simulink library "lib_accessory"  (Simulink 4.1.1)
undefined symbols (not defined in the file): acc_dcdc_eff, acc_elec_eff, acc_elec_efficiency, acc_elec_pwr, acc_mech_eff, acc_mech_pwr, acc_mech_trq, acc_sindafile, amb_tmp, cyc_mph, ess_on, fc_on, fd_ratio, gb_ratio, load_on, map_spd, max_pwr, tc_gc_to_fc_ratio, time_step, vc_idle_bool, vc_idle_spd, vinf, wh_radius
libraries: lib_accessory x47, lib_cosimulation x29, lib_outputs x11, simulink3 x4, sub_lib_models x2
(part 3 of 3)

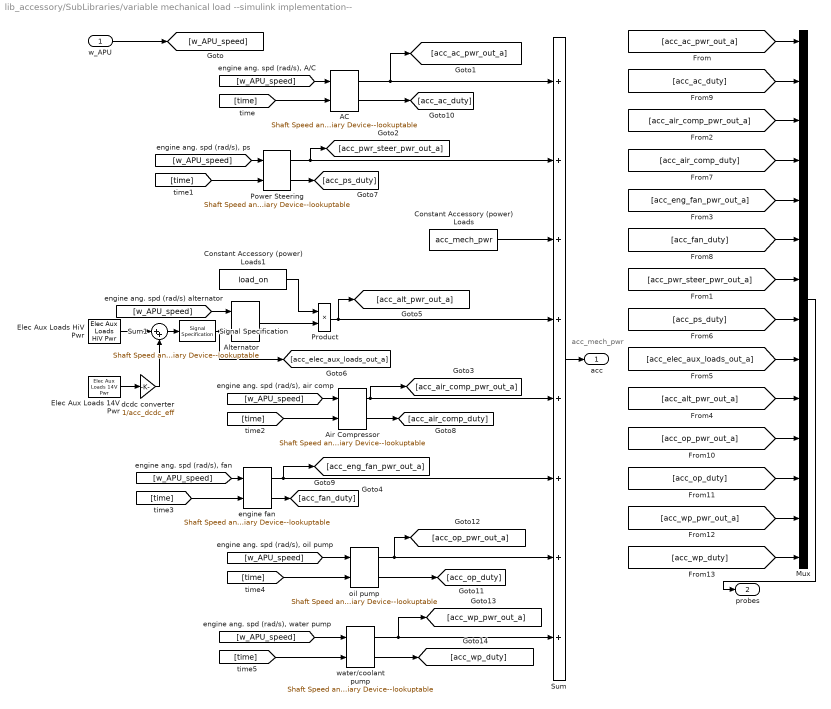
== system lib_accessory/SubLibraries/variable mechanical load --simulink implementation-- ==
  note: acc_mech_pwr
  w_APU : Inport  Port=1  LatchInput=off
  AC : lib_accessory/SubLibraries/Shaft Speed and Time Loaded Auxiliary Device--lookuptable  fname=acc_ac_init  acc_duty=acc_ac_dutycycle
  Air Compressor : lib_accessory/SubLibraries/Shaft Speed and Time Loaded Auxiliary Device--lookuptable  fname=acc_abc_init  acc_duty=acc_abc_dutycycle
  Alternator : lib_accessory/SubLibraries/Shaft Speed and Actual Load Auxiliary Device--lookuptable  conv_eff=acc_acdc_inverter_eff  fname=acc_alt_init
  Constant Accessory (power) Loads : Constant  Value=acc_mech_pwr
  Constant Accessory (power) Loads1 : Constant  Value=load_on
  Elec Aux Loads 14V Pwr : lib_accessory/Elec Aux Loads 14V Pwr
      settings: RTWFcnNameOpts=Auto  RTWFileNameOpts=Auto
  Elec Aux Loads HiV Pwr : lib_accessory/Elec Aux Loads HiV Pwr
      settings: RTWFcnNameOpts=Auto  RTWFileNameOpts=Auto
  Mux : Mux  Inputs=14
  Power Steering : lib_accessory/SubLibraries/Shaft Speed and Time Loaded Auxiliary Device--lookuptable  fname=acc_ps_init  acc_duty=acc_ps_dutycycle
  Product : Product  Inputs=2  Multiplication=Element-wise(.*)  SaturateOnIntegerOverflow=on
  Signal Specification : simulink3/Signals & Systems/Signal Specification  D=1  Ts=-1  DataType=auto
  Sum : Sum  Inputs=++++++++  SaturateOnIntegerOverflow=on
  Sum1 : Sum  Inputs=|++  SaturateOnIntegerOverflow=on
  dcdc converter : Gain  Gain=1/acc_dcdc_eff  Multiplication=Element-wise(K.*u)  SaturateOnIntegerOverflow=on
  engine fan : lib_accessory/SubLibraries/Shaft Speed and Time Loaded Auxiliary Device--lookuptable  fname=acc_ef_init  acc_duty=acc_ef_dutycycle
  oil pump : lib_accessory/SubLibraries/Shaft Speed and Time Loaded Auxiliary Device--lookuptable  fname=acc_op_init  acc_duty=acc_op_dutycycle
  water/coolant pump : lib_accessory/SubLibraries/Shaft Speed and Time Loaded Auxiliary Device--lookuptable  fname=acc_wp_init  acc_duty=acc_wp_dutycycle
  acc : Outport  Port=1
  probes : Outport  Port=2
  wires:
  [time] -> AC/2
  [w_APU_speed] -> AC/1
  AC/2 -> [acc_ac_duty]
  AC/1 -> Sum/1, [acc_ac_pwr_out_a]
  Constant Accessory (power) Loads/1 -> Sum/3
  Sum/1 -> acc/1
  [w_APU_speed] -> Alternator/1
  Air Compressor/2 -> [acc_air_comp_duty]
  Air Compressor/1 -> Sum/5, [acc_air_comp_pwr_out_a]
  [w_APU_speed] -> Air Compressor/1
  [time] -> Air Compressor/2
  oil pump/1 -> [acc_op_pwr_out_a], Sum/7
  oil pump/2 -> [acc_op_duty]
  [time] -> oil pump/2
  [w_APU_speed] -> oil pump/1
  engine fan/2 -> [acc_fan_duty]
  [time] -> engine fan/2
  engine fan/1 -> Sum/6, [acc_eng_fan_pwr_out_a]
  [w_APU_speed] -> engine fan/1
  Power Steering/2 -> [acc_ps_duty]
  [w_APU_speed] -> Power Steering/1
  [time] -> Power Steering/2
  Power Steering/1 -> Sum/2, [acc_pwr_steer_pwr_out_a]
  w_APU/1 -> [w_APU_speed]
  Elec Aux Loads 14V Pwr/1 -> dcdc converter/1
  Signal Specification/1 -> Alternator/2, [acc_elec_aux_loads_out_a]
  [acc_ac_pwr_out_a] -> Mux/1
  Product/1 -> Sum/4, [acc_alt_pwr_out_a]
  Constant Accessory (power) Loads1/1 -> Product/1
  Alternator/1 -> Product/2
  Mux/1 -> probes/1
  water/coolant pump/1 -> Sum/8, [acc_wp_pwr_out_a]
  [time] -> water/coolant pump/2
  [w_APU_speed] -> water/coolant pump/1
  water/coolant pump/2 -> [acc_wp_duty]
  [acc_ac_duty] -> Mux/2
  [acc_air_comp_pwr_out_a] -> Mux/3
  [acc_air_comp_duty] -> Mux/4
  [acc_eng_fan_pwr_out_a] -> Mux/5
  [acc_fan_duty] -> Mux/6
  [acc_pwr_steer_pwr_out_a] -> Mux/7
  [acc_ps_duty] -> Mux/8
  [acc_elec_aux_loads_out_a] -> Mux/9
  [acc_alt_pwr_out_a] -> Mux/10
  [acc_op_pwr_out_a] -> Mux/11
  [acc_op_duty] -> Mux/12
  [acc_wp_pwr_out_a] -> Mux/13
  [acc_wp_duty] -> Mux/14
  Sum1/1 -> Signal Specification/1
  Elec Aux Loads HiV Pwr/1 -> Sum1/1
  dcdc converter/1 -> Sum1/2

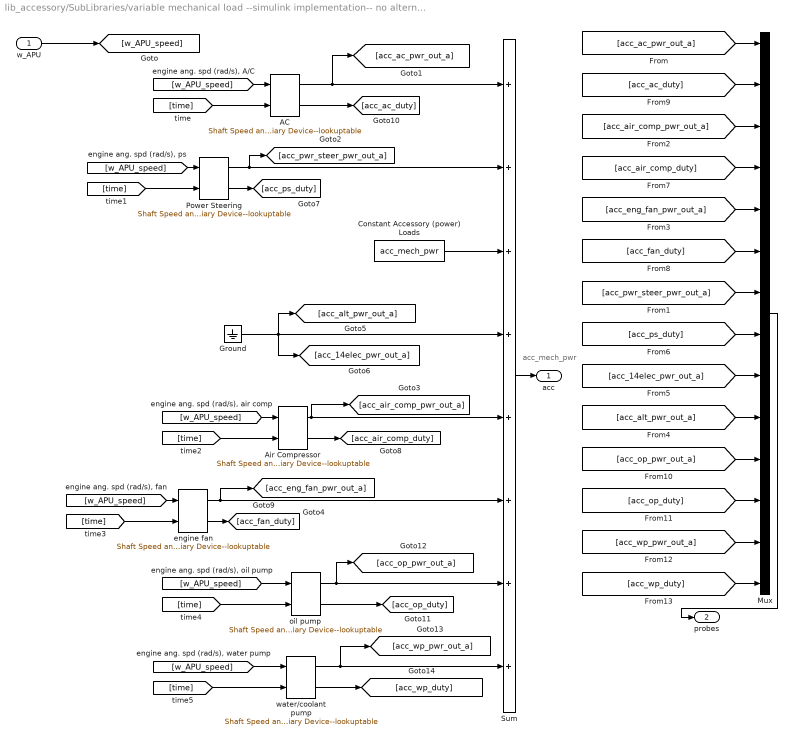
== system lib_accessory/SubLibraries/variable mechanical load --simulink implementation-- no alternator ==
  note: acc_mech_pwr
  w_APU : Inport  Port=1  LatchInput=off
  AC : lib_accessory/SubLibraries/Shaft Speed and Time Loaded Auxiliary Device--lookuptable  fname=acc_ac_init  acc_duty=acc_ac_dutycycle
  Air Compressor : lib_accessory/SubLibraries/Shaft Speed and Time Loaded Auxiliary Device--lookuptable  fname=acc_abc_init  acc_duty=acc_abc_dutycycle
  Constant Accessory (power) Loads : Constant  Value=acc_mech_pwr
  Ground : Ground
  Mux : Mux  Inputs=14
  Power Steering : lib_accessory/SubLibraries/Shaft Speed and Time Loaded Auxiliary Device--lookuptable  fname=acc_ps_init  acc_duty=acc_ps_dutycycle
  Sum : Sum  Inputs=++++++++  SaturateOnIntegerOverflow=on
  engine fan : lib_accessory/SubLibraries/Shaft Speed and Time Loaded Auxiliary Device--lookuptable  fname=acc_ef_init  acc_duty=acc_ef_dutycycle
  oil pump : lib_accessory/SubLibraries/Shaft Speed and Time Loaded Auxiliary Device--lookuptable  fname=acc_op_init  acc_duty=acc_op_dutycycle
  water/coolant pump : lib_accessory/SubLibraries/Shaft Speed and Time Loaded Auxiliary Device--lookuptable  fname=acc_wp_init  acc_duty=acc_wp_dutycycle
  acc : Outport  Port=1
  probes : Outport  Port=2
  wires:
  [time] -> AC/2
  [w_APU_speed] -> AC/1
  AC/2 -> [acc_ac_duty]
  AC/1 -> Sum/1, [acc_ac_pwr_out_a]
  Constant Accessory (power) Loads/1 -> Sum/3
  Sum/1 -> acc/1
  Air Compressor/2 -> [acc_air_comp_duty]
  Air Compressor/1 -> Sum/5, [acc_air_comp_pwr_out_a]
  [w_APU_speed] -> Air Compressor/1
  [time] -> Air Compressor/2
  oil pump/1 -> [acc_op_pwr_out_a], Sum/7
  oil pump/2 -> [acc_op_duty]
  [time] -> oil pump/2
  [w_APU_speed] -> oil pump/1
  engine fan/2 -> [acc_fan_duty]
  [time] -> engine fan/2
  engine fan/1 -> Sum/6, [acc_eng_fan_pwr_out_a]
  [w_APU_speed] -> engine fan/1
  Power Steering/2 -> [acc_ps_duty]
  [w_APU_speed] -> Power Steering/1
  [time] -> Power Steering/2
  Power Steering/1 -> Sum/2, [acc_pwr_steer_pwr_out_a]
  w_APU/1 -> [w_APU_speed]
  [acc_ac_pwr_out_a] -> Mux/1
  Ground/1 -> Sum/4, [acc_alt_pwr_out_a], [acc_14elec_pwr_out_a]
  Mux/1 -> probes/1
  water/coolant pump/1 -> Sum/8, [acc_wp_pwr_out_a]
  [time] -> water/coolant pump/2
  [w_APU_speed] -> water/coolant pump/1
  water/coolant pump/2 -> [acc_wp_duty]
  [acc_ac_duty] -> Mux/2
  [acc_air_comp_pwr_out_a] -> Mux/3
  [acc_air_comp_duty] -> Mux/4
  [acc_eng_fan_pwr_out_a] -> Mux/5
  [acc_fan_duty] -> Mux/6
  [acc_pwr_steer_pwr_out_a] -> Mux/7
  [acc_ps_duty] -> Mux/8
  [acc_14elec_pwr_out_a] -> Mux/9
  [acc_alt_pwr_out_a] -> Mux/10
  [acc_op_pwr_out_a] -> Mux/11
  [acc_op_duty] -> Mux/12
  [acc_wp_pwr_out_a] -> Mux/13
  [acc_wp_duty] -> Mux/14

== system lib_accessory/Development/Electrical Accessory Loads <acc>/Accessory SDO ==
  data bus : Inport  Port=1  LatchInput=off
  Demux : Demux  Outputs=3  BusSelectionMode=off
  To Workspace : ToWorkspace  VariableName=acc_elec_pwr_r  SampleTime=-1  SaveFormat=Array
  To Workspace3 : ToWorkspace  VariableName=acc_elec_pwr_a  SampleTime=-1  SaveFormat=Array
  To Workspace4 : ToWorkspace  VariableName=acc_elec_pwr_est  SampleTime=-1  SaveFormat=Array
  electrical power logging : lib_accessory/SubLibraries/electrical power logging  eff=acc_mech_eff
  wires:
  data bus/1 -> Demux/1
  Demux/1 -> To Workspace/1
  Demux/2 -> To Workspace3/1, electrical power logging/1
  Demux/3 -> To Workspace4/1

== system lib_accessory/Development/Electrical Accessory Loads <acc>/Block NOTES ==
  note: In terms of an interface, the model assumes electrical power generated from
      | a powersource (or powersources)
      |
      | This model takes in requested driveline electrical power output requests and
      | augments power to account for electrically driven accessories.
      |
      | The power passed along down to the driveline is only power to move the
      | vehicle.
  note: This is the electrical auxiliary loads model.

== system lib_accessory/Development/Electrical Accessory Loads <acc>/backward model ==
  note: Pwr, W, powersource out
  note: P, W, for driveline
  note: Power Electrical
      | Accessory
      | (W)
  pwr_in : Inport  Port=1  LatchInput=off
  Sum : Sum  Inputs=|++  SaturateOnIntegerOverflow=on
  electrical accessories (W) : Subsystem  BlockChoice=Electrical Accessories: Time Variable
      settings: AttributesFormatString=%<BlockChoice>  TemplateBlock=lib_accessory/electrical accessories (W)  MemberBlocks=Electrical Accessories: Constant,Electrical Accessories: Time Variable  RTWFcnNameOpts=Auto  RTWFileNameOpts=Auto
      mask Display: image(imread('bdi_acc_elec.bmp'))
  elec_out : Outport  Port=1
  elec_acc_out : Outport  Port=2
  wires:
  electrical accessories (W)/1(P_elec_acc) -> elec_acc_out/1, Sum/2
  Sum/1 -> elec_out/1
  pwr_in/1 -> Sum/1

== system lib_accessory/Development/Electrical Accessory Loads <acc>/forward model ==
  note: Power to driveline
  note: Power Available
  note: electric
      | accessory
      | power (W)
  pwr_in : Inport  Port=1  LatchInput=off
  Sum : Sum  Inputs=|+-  SaturateOnIntegerOverflow=on
  electrical accessories (W) : Subsystem  BlockChoice=Electrical Accessories: Time Variable
      settings: AttributesFormatString=%<BlockChoice>  TemplateBlock=lib_accessory/electrical accessories (W)  MemberBlocks=Electrical Accessories: Constant,Electrical Accessories: Time Variable  RTWFcnNameOpts=Auto  RTWFileNameOpts=Auto
      mask Display: image(imread('bdi_acc_elec.bmp'))
  pwr_out : Outport  Port=1
  acc_pwr_out : Outport  Port=2
  wires:
  electrical accessories (W)/1(P_elec_acc) -> acc_pwr_out/1, Sum/2
  Sum/1 -> pwr_out/1
  pwr_in/1 -> Sum/1

== system lib_accessory/Development/Mechanical Accessory Loads <acc>/Accessory SDO ==
  data bus : Inport  Port=1  LatchInput=off
  Demux : Demux  Outputs=5  BusSelectionMode=off
  To Workspace : ToWorkspace  VariableName=acc_mech_trq_r  SampleTime=-1  SaveFormat=Array
  To Workspace1 : ToWorkspace  VariableName=acc_mech_pwr_a  SampleTime=-1  SaveFormat=Array
  To Workspace2 : ToWorkspace  VariableName=acc_mech_trq_est  SampleTime=-1  SaveFormat=Array
  To Workspace3 : ToWorkspace  VariableName=acc_mech_pwr_r  SampleTime=-1  SaveFormat=Array
  To Workspace4 : ToWorkspace  VariableName=acc_mech_trq_a  SampleTime=-1  SaveFormat=Array
  mechanical power logging : lib_accessory/SubLibraries/mechanical power logging  eff=acc_mech_eff
  wires:
  data bus/1 -> Demux/1
  Demux/4 -> mechanical power logging/1, To Workspace1/1
  Demux/1 -> To Workspace/1
  Demux/2 -> To Workspace3/1
  Demux/3 -> To Workspace4/1
  Demux/5 -> To Workspace2/1

== system lib_accessory/Development/Mechanical Accessory Loads <acc>/Block NOTES ==
  note: This is the mechanical auxiliary loads model.
  note: In terms of an interface, the model assumes belt-driven mechanical loads
      | that run off of a prime mover shaft (e.g., engine shaft)
      |
      | This model takes in requested driveline torque and speed requests and
      | augments torque due to belt driven accessories.
      |
      | The torque passed along down to the driveline is only torque to move the
      | vehicle.

== system lib_accessory/Development/Mechanical Accessory Loads <acc>/backward model ==
  note: w_apu, rad/s
  note: T, Nm, accessory
  note: T, Nm, driveline
  note: T, Nm, shaft out
  note: Power, W, input to accessory
  trq_in : Inport  Port=1  LatchInput=off
  spd_in : Inport  Port=2  LatchInput=off
  Sum : Sum  Inputs=|++  SaturateOnIntegerOverflow=on
  mechanical accessories (Nm) : Subsystem  BlockChoice=Mechanical Accessories: Const Mech Var Elect
      settings: AttributesFormatString=%<BlockChoice>  TemplateBlock=lib_accessory/mechanical accessories (Nm)  MemberBlocks=Mechanical Accessories: Const Mech Var Elect,Mechanical Accessories: Constant Load No Alternator,Mechanical Accessories: Constant Mechanical & Electrical,Mechanical Accessories: Speed Dependant No Alternator,Mechanical Accessories: Speed Dependant and Variable Electrical  RTWFcnNameOpts=Auto  RTWFileNameOpts=Auto
      mask Display: image(imread('bdi_acc_pic.bmp'))
  trq_out : Outport  Port=1
  spd_out : Outport  Port=2
  acc_mech_trq_r : Outport  Port=3
  acc_mech_pwr_r : Outport  Port=4
  wires:
  spd_in/1 -> spd_out/1, mechanical accessories (Nm)/1(w_APU)
  mechanical accessories (Nm)/1(T_acc) -> acc_mech_trq_r/1, Sum/2
  trq_in/1 -> Sum/1
  Sum/1 -> trq_out/1
  mechanical accessories (Nm)/2(P_mech_acc) -> acc_mech_pwr_r/1

== system lib_accessory/Development/Mechanical Accessory Loads <acc>/estimated mechanical torque ==
  spd_in : Inport  Port=1  LatchInput=off
  mech pwr : Terminator
  mechanical accessories (Nm) : Subsystem  BlockChoice=Mechanical Accessories: Const Mech Var Elect
      settings: AttributesFormatString=%<BlockChoice>  TemplateBlock=lib_accessory/mechanical accessories (Nm)  MemberBlocks=Mechanical Accessories: Const Mech Var Elect,Mechanical Accessories: Constant Load No Alternator,Mechanical Accessories: Constant Mechanical & Electrical,Mechanical Accessories: Speed Dependant No Alternator,Mechanical Accessories: Speed Dependant and Variable Electrical  RTWFcnNameOpts=Auto  RTWFileNameOpts=Auto
      mask Display: image(imread('bdi_acc_pic.bmp'))
  trq_out : Outport  Port=1
  wires:
  spd_in/1 -> mechanical accessories (Nm)/1(w_APU)
  mechanical accessories (Nm)/2(P_mech_acc) -> mech pwr/1
  mechanical accessories (Nm)/1(T_acc) -> trq_out/1

== system lib_accessory/Development/Mechanical Accessory Loads <acc>/forward model ==
  note: w_apu, rad/s
  note: T, Nm, accessory
  note: T, Nm, driveline
  note: T, Nm, shaft out
  note: Power, W, input to accessory
  trq_in : Inport  Port=1  LatchInput=off
  spd_in : Inport  Port=2  LatchInput=off
  Sum : Sum  Inputs=|+-  SaturateOnIntegerOverflow=on
  mechanical accessories (Nm) : Subsystem  BlockChoice=Mechanical Accessories: Const Mech Var Elect
      settings: AttributesFormatString=%<BlockChoice>  TemplateBlock=lib_accessory/mechanical accessories (Nm)  MemberBlocks=Mechanical Accessories: Const Mech Var Elect,Mechanical Accessories: Constant Load No Alternator,Mechanical Accessories: Constant Mechanical & Electrical,Mechanical Accessories: Speed Dependant No Alternator,Mechanical Accessories: Speed Dependant and Variable Electrical  RTWFcnNameOpts=Auto  RTWFileNameOpts=Auto
      mask Display: image(imread('bdi_acc_pic.bmp'))
  trq_out : Outport  Port=1
  spd_out : Outport  Port=2
  acc_mech_trq_a : Outport  Port=3
  acc_mech_pwr_a : Outport  Port=4
  wires:
  spd_in/1 -> spd_out/1, mechanical accessories (Nm)/1(w_APU)
  mechanical accessories (Nm)/1(T_acc) -> acc_mech_trq_a/1, Sum/2
  trq_in/1 -> Sum/1
  Sum/1 -> trq_out/1
  mechanical accessories (Nm)/2(P_mech_acc) -> acc_mech_pwr_a/1

== system lib_accessory/Elec Aux Loads HiV Pwr/Starter/Starter ==
  14 V : Constant  Value=vinf.AuxLoads.Starter.HiV
  Hit  Crossing : HitCross  HitCrossingOffset=0  HitCrossingDirection=rising  ShowOutputPort=on
  Memory : Memory  X0=fc_on  InheritSampleTime=off
      settings: RTWStateStorageClass=Auto
  On : Constant  Value=vinf.AuxLoads.Starter.On
  Product1 : Product  Inputs=4  Multiplication=Element-wise(.*)  SaturateOnIntegerOverflow=on
  Subsystem : Subsystem
      settings: RTWFcnNameOpts=Auto  RTWFileNameOpts=Auto
  Starter_OnOff_Control : Outport  Port=1
  wires:
  14 V/1 -> Product1/2
  Subsystem/1(Out1) -> Product1/3
  Product1/1 -> Starter_OnOff_Control/1
  On/1 -> Product1/1
  [key_on] -> Product1/4
  [time] -> Subsystem/2(In2)
  [engine_on] -> Memory/1
  Hit  Crossing/1 -> Subsystem/1(In1)
  Memory/1 -> Hit  Crossing/1

== system lib_accessory/Electrical Accessory Loads v2 <acc>/backward model/electrical accessories (W) ==
  Electrical Accessories: Time Variable : lib_accessory/Electrical Accessories: Time Variable
  P_elec_acc : Outport  Port=1
  wires:
  Electrical Accessories: Time Variable/1 -> P_elec_acc/1

== system lib_accessory/Mechanical Accessory Loads v2 <acc>/backward model/mechanical accessories (Nm) ==
  w_APU : Inport  Port=1  LatchInput=off
  Mechanical Accessories: Const Mech Var Elect : lib_accessory/Mechanical Accessories: Const Mech Var Elect
  T_acc : Outport  Port=1
  P_mech_acc : Outport  Port=2
  probes : Outport  Port=3
  wires:
  w_APU/1 -> Mechanical Accessories: Const Mech Var Elect/1
  Mechanical Accessories: Const Mech Var Elect/1 -> T_acc/1
  Mechanical Accessories: Const Mech Var Elect/2 -> P_mech_acc/1
  Mechanical Accessories: Const Mech Var Elect/3 -> probes/1

== system lib_accessory/Saber Dual Voltage Cosim/saber dv acc/DV cosim output gotos ==
  In1 : Inport  Port=1  LatchInput=off
  Demux : Demux  Outputs=[4 4 4 2 2 30 12]  BusSelectionMode=off
  Saber_ess2_outputs : Subsystem  BlockChoice=Saber_rint2
      settings: AttributesFormatString=%<BlockChoice>  TemplateBlock=lib_outputs/Saber_ess2_outputs  MemberBlocks=Saber_pb2,Saber_rint2  RTWFcnNameOpts=Auto  RTWFileNameOpts=Auto
  Saber_ess_outputs : Subsystem  BlockChoice=Saber_rint
      settings: AttributesFormatString=%<BlockChoice>  TemplateBlock=lib_outputs/Saber_ess_outputs  MemberBlocks=Saber_pb,Saber_rint  RTWFcnNameOpts=Auto  RTWFileNameOpts=Auto
  saber acc 14v output gotos : lib_outputs/saber acc 14v output gotos
      settings: RTWFcnNameOpts=Auto  RTWFileNameOpts=Auto
  saber acc HiV output gotos : lib_outputs/saber acc HiV output gotos
      settings: RTWFcnNameOpts=Auto  RTWFileNameOpts=Auto
  saber acc additional outputs : lib_outputs/saber acc additional outputs
      settings: RTWFcnNameOpts=Auto  RTWFileNameOpts=Auto
  saber dcdc output gotos : lib_outputs/saber dcdc output gotos
      settings: RTWFcnNameOpts=Auto  RTWFileNameOpts=Auto
  saber gc output gotos : lib_outputs/saber gc output gotos
      settings: RTWFcnNameOpts=Auto  RTWFileNameOpts=Auto
  Out1 : Outport  Port=1
  wires:
  Demux/3 -> Saber_ess2_outputs/1(In1)
  Demux/2 -> Saber_ess_outputs/1(In1)
  In1/1 -> Demux/1
  Demux/1 -> saber gc output gotos/1
  Demux/4 -> saber dcdc output gotos/1
  saber gc output gotos/1 -> Out1/1
  Demux/6 -> saber acc 14v output gotos/1
  Demux/7 -> saber acc HiV output gotos/1
  Demux/5 -> saber acc additional outputs/1

== system lib_accessory/Saber Dual Voltage Cosim/saber dv acc/Engine Info ==
  w_apu : Inport  Port=1  LatchInput=off
  Constant : Constant  Value=0
  Enabled Subsystem : Subsystem  TreatAsAtomicUnit=on
      settings: RTWFcnNameOpts=Auto  RTWFileNameOpts=Auto
  IC : InitialCondition  Value=time_step
  Matrix Concatenation1 : S-Function  FunctionName=smatrxcat  Parameters=numInports,catMethod  PortCounts=[]  SFunctionModules=''  mask(Matrix Concatenation){numInports=6, catMethod=Horizontal}
      mask prompts: numInports "Number of inputs:"; catMethod "Concatenation method:"
      mask help: Perform horizontal or vertical concatenation. 1-D vector input signals are treated as column vectors, i.e., [Mx1] matrices. The output is always a matrix.
      mask init:
      | xy = matrxcatmask('icon');
      mask StyleString: edit,popup(Horizontal|Vertical)
      mask Display:
      | plot(xy.x,xy.y);
      | text(0.15,0.86,xy.label);
  Memory1 : Memory  X0=.001  InheritSampleTime=on
      settings: RTWStateStorageClass=Auto
  Memory2 : Memory  X0=80  InheritSampleTime=on
      settings: RTWStateStorageClass=Auto
  Relational Operator : RelationalOperator  Operator===
  Saturation : Saturate  UpperLimit=inf  LowerLimit=.001  LinearizeAsGain=on
  pulley ratio : Gain  Gain=tc_gc_to_fc_ratio  Multiplication=Element-wise(K.*u)  SaturateOnIntegerOverflow=on
  "rad/s -> rpm1" : Gain  Gain=60/(2*pi)  Multiplication=Element-wise(K.*u)  SaturateOnIntegerOverflow=on
  RPM : Outport  Port=1
  wires:
  Relational Operator/1 -> Enabled Subsystem/Enable
  [time] -> Relational Operator/2
  Enabled Subsystem/1(Out1) -> Matrix Concatenation1/2
  Memory2/1 -> Matrix Concatenation1/4
  Matrix Concatenation1/1 -> RPM/1
  IC/1 -> Matrix Concatenation1/5
  Saturation/1 -> Memory1/1
  [time] -> Saturation/1
  Memory1/1 -> Matrix Concatenation1/3
  [time] -> IC/1
  Constant/1 -> Relational Operator/1, Matrix Concatenation1/1
  w_apu/1 -> "rad/s -> rpm1"/1  "w_apu"
  "rad/s -> rpm1"/1 -> pulley ratio/1
  pulley ratio/1 -> Enabled Subsystem/1(In1), Matrix Concatenation1/6, Memory2/1

== system lib_accessory/Saber Dual Voltage Cosim/saber dv acc/Model Data In ==
  Aux Loads 14V and 42V : Subsystem
      settings: RTWFcnNameOpts=Auto  RTWFileNameOpts=Auto
  DC/DC converter : lib_cosimulation/DC//DC converter
      settings: RTWFcnNameOpts=Auto  RTWFileNameOpts=Auto
  Generator : lib_cosimulation/Generator
      settings: RTWFcnNameOpts=Auto  RTWFileNameOpts=Auto
  Matrix Concatenation1 : S-Function  FunctionName=smatrxcat  Parameters=numInports,catMethod  PortCounts=[]  SFunctionModules=''  mask(Matrix Concatenation){numInports=6, catMethod=Horizontal}
      mask prompts: numInports "Number of inputs:"; catMethod "Concatenation method:"
      mask help: Perform horizontal or vertical concatenation. 1-D vector input signals are treated as column vectors, i.e., [Mx1] matrices. The output is always a matrix.
      mask init:
      | xy = matrxcatmask('icon');
      mask StyleString: edit,popup(Horizontal|Vertical)
      mask Display:
      | plot(xy.x,xy.y);
      | text(0.15,0.86,xy.label);
  Regulator : lib_cosimulation/Regulator
      settings: RTWFcnNameOpts=Auto  RTWFileNameOpts=Auto
  ess param inputs : Subsystem  BlockChoice=Rint
      settings: AttributesFormatString=%<BlockChoice>  TemplateBlock=lib_cosimulation/ess param inputs  MemberBlocks=Rint,Saber lib pb  RTWFcnNameOpts=Auto  RTWFileNameOpts=Auto
  ess2 param inputs : Subsystem  BlockChoice=Rint2
      settings: AttributesFormatString=%<BlockChoice>  TemplateBlock=lib_cosimulation/ess2 param inputs  MemberBlocks=Rint2,Saber lib pb2  RTWFcnNameOpts=Auto  RTWFileNameOpts=Auto
  Out1 : Outport  Port=1
  wires:
  Aux Loads 14V and 42V/1(Out1) -> Matrix Concatenation1/1
  Regulator/1 -> Matrix Concatenation1/4
  Matrix Concatenation1/1 -> Out1/1
  Generator/1 -> Matrix Concatenation1/2
  DC/DC converter/1 -> Matrix Concatenation1/3
  ess param inputs/1(Out1) -> Matrix Concatenation1/5
  ess2 param inputs/1(Out1) -> Matrix Concatenation1/6

== system lib_accessory/Saber Single Voltage Cosim/saber sv acc/Engine Info ==
  w_apu : Inport  Port=1  LatchInput=off
  Constant : Constant  Value=0
  Enabled Subsystem : Subsystem  TreatAsAtomicUnit=on
      settings: RTWFcnNameOpts=Auto  RTWFileNameOpts=Auto
  IC : InitialCondition  Value=time_step
  Matrix Concatenation1 : S-Function  FunctionName=smatrxcat  Parameters=numInports,catMethod  PortCounts=[]  SFunctionModules=''  mask(Matrix Concatenation){numInports=6, catMethod=Horizontal}
      mask prompts: numInports "Number of inputs:"; catMethod "Concatenation method:"
      mask help: Perform horizontal or vertical concatenation. 1-D vector input signals are treated as column vectors, i.e., [Mx1] matrices. The output is always a matrix.
      mask init:
      | xy = matrxcatmask('icon');
      mask StyleString: edit,popup(Horizontal|Vertical)
      mask Display:
      | plot(xy.x,xy.y);
      | text(0.15,0.86,xy.label);
  Memory1 : Memory  X0=.001  InheritSampleTime=on
      settings: RTWStateStorageClass=Auto
  Memory2 : Memory  X0=80  InheritSampleTime=on
      settings: RTWStateStorageClass=Auto
  Relational Operator : RelationalOperator  Operator===
  Saturation : Saturate  UpperLimit=inf  LowerLimit=.001  LinearizeAsGain=on
  pulley ratio : Gain  Gain=tc_gc_to_fc_ratio  Multiplication=Element-wise(K.*u)  SaturateOnIntegerOverflow=on
  "rad/s -> rpm1" : Gain  Gain=60/(2*pi)  Multiplication=Element-wise(K.*u)  SaturateOnIntegerOverflow=on
  RPM : Outport  Port=1
  wires:
  Relational Operator/1 -> Enabled Subsystem/Enable
  [time] -> Relational Operator/2
  Enabled Subsystem/1(Out1) -> Matrix Concatenation1/2
  Memory2/1 -> Matrix Concatenation1/4
  Matrix Concatenation1/1 -> RPM/1
  IC/1 -> Matrix Concatenation1/5
  Saturation/1 -> Memory1/1
  [time] -> Saturation/1
  Memory1/1 -> Matrix Concatenation1/3
  [time] -> IC/1
  Constant/1 -> Relational Operator/1, Matrix Concatenation1/1
  w_apu/1 -> "rad/s -> rpm1"/1  "w_apu"
  "rad/s -> rpm1"/1 -> pulley ratio/1
  pulley ratio/1 -> Enabled Subsystem/1(In1), Matrix Concatenation1/6, Memory2/1

== system lib_accessory/Saber Single Voltage Cosim/saber sv acc/SV Model Data In ==
  Aux Loads 14V : lib_cosimulation/Aux Loads 14V
      settings: RTWFcnNameOpts=Auto  RTWFileNameOpts=Auto
  Elec Aux Loads Additional : lib_cosimulation/Elec Aux Loads Additional
      settings: RTWFcnNameOpts=Auto  RTWFileNameOpts=Auto
  Generator : lib_cosimulation/Generator
      settings: RTWFcnNameOpts=Auto  RTWFileNameOpts=Auto
  Matrix Concatenation1 : S-Function  FunctionName=smatrxcat  Parameters=numInports,catMethod  PortCounts=[]  SFunctionModules=''  mask(Matrix Concatenation){numInports=5, catMethod=Horizontal}
      mask prompts: numInports "Number of inputs:"; catMethod "Concatenation method:"
      mask help: Perform horizontal or vertical concatenation. 1-D vector input signals are treated as column vectors, i.e., [Mx1] matrices. The output is always a matrix.
      mask init:
      | xy = matrxcatmask('icon');
      mask StyleString: edit,popup(Horizontal|Vertical)
      mask Display:
      | plot(xy.x,xy.y);
      | text(0.15,0.86,xy.label);
  Regulator : lib_cosimulation/Regulator
      settings: RTWFcnNameOpts=Auto  RTWFileNameOpts=Auto
  ess2 param inputs : Subsystem  BlockChoice=Rint2
      settings: AttributesFormatString=%<BlockChoice>  TemplateBlock=lib_cosimulation/ess2 param inputs  MemberBlocks=Rint2,Saber lib pb2  RTWFcnNameOpts=Auto  RTWFileNameOpts=Auto
  Out1 : Outport  Port=1
  wires:
  Matrix Concatenation1/1 -> Out1/1
  ess2 param inputs/1(Out1) -> Matrix Concatenation1/5
  Regulator/1 -> Matrix Concatenation1/4
  Generator/1 -> Matrix Concatenation1/3
  Elec Aux Loads Additional/1 -> Matrix Concatenation1/1
  Aux Loads 14V/1 -> Matrix Concatenation1/2

== system lib_accessory/Saber Single Voltage Cosim/saber sv acc/SV cosim output gotos ==
  In1 : Inport  Port=1  LatchInput=off
  Demux : Demux  Outputs=[4 4 2 30]  BusSelectionMode=off
  Saber_ess2_outputs : Subsystem  BlockChoice=Saber_rint2
      settings: AttributesFormatString=%<BlockChoice>  TemplateBlock=lib_outputs/Saber_ess2_outputs  MemberBlocks=Saber_pb2,Saber_rint2  RTWFcnNameOpts=Auto  RTWFileNameOpts=Auto
  saber acc 14v output gotos : lib_outputs/saber acc 14v output gotos
      settings: RTWFcnNameOpts=Auto  RTWFileNameOpts=Auto
  saber acc additional outputs : lib_outputs/saber acc additional outputs
      settings: RTWFcnNameOpts=Auto  RTWFileNameOpts=Auto
  saber gc output gotos : lib_outputs/saber gc output gotos
      settings: RTWFcnNameOpts=Auto  RTWFileNameOpts=Auto
  Out1 : Outport  Port=1
  wires:
  Demux/2 -> Saber_ess2_outputs/1(In1)
  Demux/1 -> saber gc output gotos/1
  In1/1 -> Demux/1
  saber gc output gotos/1 -> Out1/1
  Demux/4 -> saber acc 14v output gotos/1
  Demux/3 -> saber acc additional outputs/1

== system lib_accessory/SubLibraries/Shaft Speed and Time Loaded Auxiliary Device/device duty  schedule by time ==
  distance travelled (m) : Inport  Port=1  LatchInput=off
  Fcn1 : Fcn  Expr=rem(u[1],period)
  Look-Up Table : Lookup  InputValues=t  OutputValues=y
  out_1 : Outport  Port=1  InitialOutput=0
  wires:
  Look-Up Table/1 -> out_1/1
  Fcn1/1 -> Look-Up Table/1
  distance travelled (m)/1 -> Fcn1/1

== system lib_accessory/SubLibraries/Shaft Speed and Time Loaded Auxiliary Device--lookuptable/device duty  schedule by time ==
  distance travelled (m) : Inport  Port=1  LatchInput=off
  Fcn1 : Fcn  Expr=rem(u[1],period)
  Look-Up Table : Lookup  InputValues=t  OutputValues=y
  out_1 : Outport  Port=1  InitialOutput=0
  wires:
  distance travelled (m)/1 -> Fcn1/1
  Fcn1/1 -> Look-Up Table/1
  Look-Up Table/1 -> out_1/1

== system lib_accessory/Development/Electrical Accessory Loads <acc>/backward model/electrical accessories (W) ==
  Electrical Accessories: Time Variable : lib_accessory/Electrical Accessories: Time Variable
  P_elec_acc : Outport  Port=1
  wires:
  Electrical Accessories: Time Variable/1 -> P_elec_acc/1

== system lib_accessory/Development/Electrical Accessory Loads <acc>/forward model/electrical accessories (W) ==
  Electrical Accessories: Time Variable : lib_accessory/Electrical Accessories: Time Variable
  P_elec_acc : Outport  Port=1
  wires:
  Electrical Accessories: Time Variable/1 -> P_elec_acc/1

== system lib_accessory/Development/Mechanical Accessory Loads <acc>/backward model/mechanical accessories (Nm) ==
  w_APU : Inport  Port=1  LatchInput=off
  Mechanical Accessories: Const Mech Var Elect : lib_accessory/Mechanical Accessories: Const Mech Var Elect
  T_acc : Outport  Port=1
  P_mech_acc : Outport  Port=2
  wires:
  w_APU/1 -> Mechanical Accessories: Const Mech Var Elect/1
  Mechanical Accessories: Const Mech Var Elect/1 -> T_acc/1
  Mechanical Accessories: Const Mech Var Elect/2 -> P_mech_acc/1

== system lib_accessory/Development/Mechanical Accessory Loads <acc>/estimated mechanical torque/mechanical accessories (Nm) ==
  w_APU : Inport  Port=1  LatchInput=off
  Mechanical Accessories: Const Mech Var Elect : lib_accessory/Mechanical Accessories: Const Mech Var Elect
  T_acc : Outport  Port=1
  P_mech_acc : Outport  Port=2
  wires:
  w_APU/1 -> Mechanical Accessories: Const Mech Var Elect/1
  Mechanical Accessories: Const Mech Var Elect/1 -> T_acc/1
  Mechanical Accessories: Const Mech Var Elect/2 -> P_mech_acc/1

== system lib_accessory/Development/Mechanical Accessory Loads <acc>/forward model/mechanical accessories (Nm) ==
  w_APU : Inport  Port=1  LatchInput=off
  Mechanical Accessories: Const Mech Var Elect : lib_accessory/Mechanical Accessories: Const Mech Var Elect
  T_acc : Outport  Port=1
  P_mech_acc : Outport  Port=2
  wires:
  w_APU/1 -> Mechanical Accessories: Const Mech Var Elect/1
  Mechanical Accessories: Const Mech Var Elect/1 -> T_acc/1
  Mechanical Accessories: Const Mech Var Elect/2 -> P_mech_acc/1

== system lib_accessory/Elec Aux Loads HiV Pwr/Starter/Starter/Subsystem ==
  In1 : Inport  Port=1  LatchInput=off
  In2 : Inport  Port=2  LatchInput=off
  Constant : Constant  Value=vinf.AuxLoads.Starter.DurationOn
  Constant1 : Constant  Value=0
  Constant2 : Constant  Value=1
  Last Engine On Time : Subsystem  TreatAsAtomicUnit=on
      settings: RTWFcnNameOpts=Auto  RTWFileNameOpts=Auto
  Relational Operator : RelationalOperator  Operator=>
  Sum : Sum  Inputs=-+  SaturateOnIntegerOverflow=on
  Switch : Switch  Threshold=.5
  Out1 : Outport  Port=1
  wires:
  Constant/1 -> Relational Operator/1
  Sum/1 -> Relational Operator/2
  In2/1 -> Sum/2, Last Engine On Time/1(In1)  "Current TIme"
  Last Engine On Time/1(Out1) -> Sum/1
  Relational Operator/1 -> Switch/2
  Constant1/1 -> Switch/3
  In1/1 -> Last Engine On Time/Trigger
  Constant2/1 -> Switch/1
  Switch/1 -> Out1/1

== system lib_accessory/Saber Dual Voltage Cosim/saber dv acc/DV cosim output gotos/Saber_ess2_outputs ==
  In1 : Inport  Port=1  LatchInput=off
  Saber_rint2 : lib_outputs/Saber_rint2
      settings: RTWFcnNameOpts=Auto  RTWFileNameOpts=Auto
  wires:
  In1/1 -> Saber_rint2/1

== system lib_accessory/Saber Dual Voltage Cosim/saber dv acc/DV cosim output gotos/Saber_ess_outputs ==
  In1 : Inport  Port=1  LatchInput=off
  Saber_rint : lib_outputs/Saber_rint
      settings: RTWFcnNameOpts=Auto  RTWFileNameOpts=Auto
  wires:
  In1/1 -> Saber_rint/1

== system lib_accessory/Saber Dual Voltage Cosim/saber dv acc/Engine Info/Enabled Subsystem ==
  In1 : Inport  Port=1  LatchInput=off
  Enable : EnablePort
  Out1 : Outport  Port=1
  wires:
  In1/1 -> Out1/1

== system lib_accessory/Saber Dual Voltage Cosim/saber dv acc/Model Data In/Aux Loads 14V and 42V ==
  Aux Loads 14V : lib_cosimulation/Aux Loads 14V
      settings: RTWFcnNameOpts=Auto  RTWFileNameOpts=Auto
  Aux Loads 42V : lib_cosimulation/Aux Loads 42V
      settings: RTWFcnNameOpts=Auto  RTWFileNameOpts=Auto
  Elec Aux Loads Additional : lib_cosimulation/Elec Aux Loads Additional
      settings: RTWFcnNameOpts=Auto  RTWFileNameOpts=Auto
  Matrix Concatenation1 : S-Function  FunctionName=smatrxcat  Parameters=numInports,catMethod  PortCounts=[]  SFunctionModules=''  mask(Matrix Concatenation){numInports=3, catMethod=Horizontal}
      mask prompts: numInports "Number of inputs:"; catMethod "Concatenation method:"
      mask help: Perform horizontal or vertical concatenation. 1-D vector input signals are treated as column vectors, i.e., [Mx1] matrices. The output is always a matrix.
      mask init:
      | xy = matrxcatmask('icon');
      mask StyleString: edit,popup(Horizontal|Vertical)
      mask Display:
      | plot(xy.x,xy.y);
      | text(0.15,0.86,xy.label);
  Out1 : Outport  Port=1
  wires:
  Matrix Concatenation1/1 -> Out1/1
  Aux Loads 42V/1 -> Matrix Concatenation1/3
  Aux Loads 14V/1 -> Matrix Concatenation1/2
  Elec Aux Loads Additional/1 -> Matrix Concatenation1/1

== system lib_accessory/Saber Dual Voltage Cosim/saber dv acc/Model Data In/ess param inputs ==
  Rint : lib_cosimulation/Rint
      settings: RTWFcnNameOpts=Auto  RTWFileNameOpts=Auto
  Out1 : Outport  Port=1
  wires:
  Rint/1 -> Out1/1

== system lib_accessory/Saber Dual Voltage Cosim/saber dv acc/Model Data In/ess2 param inputs ==
  Rint2 : lib_cosimulation/Rint2
      settings: RTWFcnNameOpts=Auto  RTWFileNameOpts=Auto
  Out1 : Outport  Port=1
  wires:
  Rint2/1 -> Out1/1

== system lib_accessory/Saber Single Voltage Cosim/saber sv acc/Engine Info/Enabled Subsystem ==
  In1 : Inport  Port=1  LatchInput=off
  Enable : EnablePort
  Out1 : Outport  Port=1
  wires:
  In1/1 -> Out1/1

== system lib_accessory/Saber Single Voltage Cosim/saber sv acc/SV Model Data In/ess2 param inputs ==
  Rint2 : lib_cosimulation/Rint2
      settings: RTWFcnNameOpts=Auto  RTWFileNameOpts=Auto
  Out1 : Outport  Port=1
  wires:
  Rint2/1 -> Out1/1

== system lib_accessory/Saber Single Voltage Cosim/saber sv acc/SV cosim output gotos/Saber_ess2_outputs ==
  In1 : Inport  Port=1  LatchInput=off
  Saber_rint2 : lib_outputs/Saber_rint2
      settings: RTWFcnNameOpts=Auto  RTWFileNameOpts=Auto
  wires:
  In1/1 -> Saber_rint2/1

== system lib_accessory/Elec Aux Loads HiV Pwr/Starter/Starter/Subsystem/Last Engine On Time ==
  In1 : Inport  Port=1  LatchInput=off
  Trigger : TriggerPort  TriggerType=rising  OutputDataType=auto
  Out1 : Outport  Port=1  InitialOutput=-100
  wires:
  In1/1 -> Out1/1
